simulink model "Sim_Saturation_iqctest1"  (Simulink 7.3)
settings: Solver=ode45  StartTime=0.0  StopTime=10.0  RelTol=1e-3
settings Model: Creator=MD710  LastModifiedBy=MD710
settings DebuggingCC: SaveWithParameterizedLinksMsg=none  SolverPrmCheckMsg=none  MultiTaskDSMMsg=warning  MultiTaskCondExecSysMsg=none  FcnCallInpInsideContextMsg=Enable All  StrictBusMsg=None
settings HardwareCC: TargetHWDeviceType=32-bit Generic
settings RTWCC: IncludeERTFirstTime=on
settings GRTTargetCC: TargetFcnLib=ansi_tfl_tmw.mat

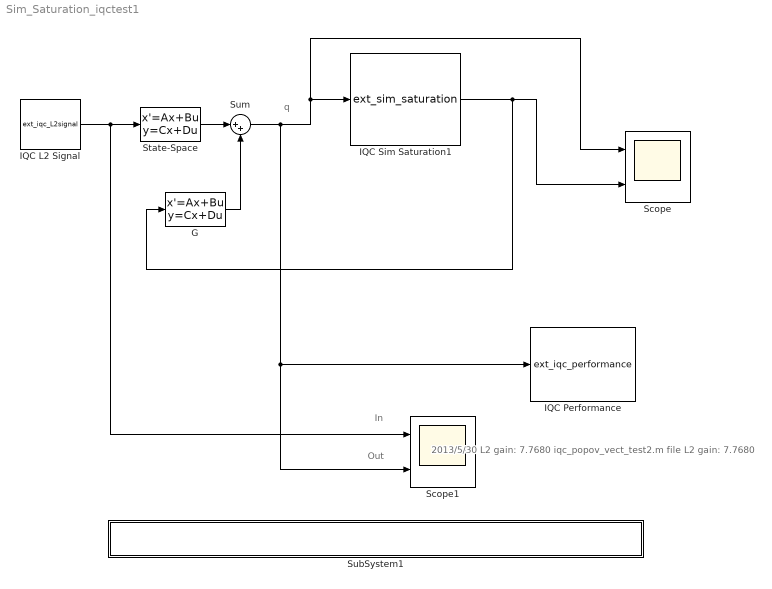
== system Sim_Saturation_iqctest1 ==
  note: q
  note: 2013/5/30 L2 gain: 7.7680
      | iqc_popov_vect_test2.m file L2 gain: 7.7680
  note: In
  note: Out
  G : StateSpace  A=[-0.37 0.20 0.15; -0.24 -0.65 0.51;0.09 -0.53 -0.60]  B="[-0.14 0; 0.11 -0.10;0   -0.83]"  C="[0.15   0    0;  0     0.8   0.4];"  D=[0 0;0 0]
  IQC L2 Signal : M-S-Function  FunctionName=ext_iqc_L2signal  Parameters=sig_size,sam_time,sig_type,tru_time,sig_amp,sig_fre,user_cus  mask(IQC L2 signal(ver:0.1)){sig_size=2, sam_time=0, sig_type=Step, tru_time=5, sig_amp=30, sig_fre=1, user_cus='2*exp(3*t)'}
      mask prompts: sig_size "Signal Dimension:(Default: 1)"; sam_time "Sample Time:(Default: 0)"; sig_type "Signal Type:"; tru_time "Truncation Time:"; sig_amp "Maximum Amplitude:"; sig_fre "Frequency:"; user_cus "Custom:"
      mask help:
      | Important:
      | In IQC procedure step (as commond iqc_gain_tbx, the task is get
      | L2 gain value), regardless of the user to choose which option (ex sine...),
      | here regarded as generalized L2 signal.
      mask StyleString: edit,edit,popup(Step|Square wave|Sine wave|Custom|Random|External),edit,edit,edit,edit
      mask CallbackString: ||iqc_block_cho(gcb,'L2signal_type')||||
      mask TabNameString: Main,Main,Simulation,Simulation,Simulation,Simulation,Simulation
      mask Display: plot(0:0.1:10,[sin(0:0.1:6.2) zeros(1,38)])
  IQC Performance : M-S-Function  FunctionName=ext_iqc_performance  Parameters=imp_met,save_lin_com,isiqcbode,fre_ran,uselmitool,lmi_par  mask(IQC Performance(ver:0.1)){imp_met=Calculation and Simulation, save_lin_com=off, isiqcbode=off, fre_ran='', uselmitool=lmilab, lmi_par=''}
      mask prompts: imp_met "Implementation Methods"; save_lin_com "Save the Linear File and Command File"; isiqcbode "Display IQC Bode Figure"; fre_ran "Frequency Range:(Default: empty)"; uselmitool "LMI Tool:"; lmi_par "Parameter:(if empty use define)"
      mask help:
      | Important:
      | In IQC toolbox calculate step (as commond iqc_gain_tbx, the task is get
      | L2 gain value), regardless of the user to connect any signal input(Even if
      | not a signal), here regarded as generalized L2 signal.
      |
      | Example 1: setlmioptions('',[0 200 0 0 777])
      | the block parameter is
      | LMI Tool: lmilab
      | Parameter:
      |        [0 200 0 0 777]
      |
      | Example 2: setlmioptions('yalmip','solver','sdpt3','verbose',1)
      | the block parameter is
      | LMI Tool: yalmip
      | Parameter:
      |        {'solver',sdpt3','verbose',1}
      mask Help:
      | <a href="matlab:doc abst_init_iqc;">abst_init_iqc</a>
      | <a href="matlab:doc setlmioptions;">setlmioptions</a>
      | <a href="matlab:doc iqc_gain_tbx;">iqc_gain_tbx</a>
      mask StyleString: popup(Calculation and Simulation|Only Calculation|Only Simulation),checkbox,checkbox,edit,popup(lmilab|yalmip),edit
      mask CallbackString: iqc_block_cho(gcb,'performance_imp')||iqc_block_cho(gcb,'performance_bodefre')|||
      mask TabNameString: Main,Main,Main,Main,LMI,LMI
      mask Display: fprintf('In -> Out \n performance \n L2 gain:\n%4.4f',7.768);
  IQC Sim Saturation1 : M-S-Function  FunctionName=ext_sim_saturation  Parameters=upp_lim,low_lim,sam_tim,iqc1,iqc1_pole,iqc1_ope,iqc1_out,iqc2,iqc2_out,iqc3,iqc3_out,iqc4,iqc4_sign,iqc4_out,iqc5,lis_rel  mask(IQC Sim Saturation(ver:0.1)){upp_lim=1, low_lim=-1, sam_tim=0, iqc1=off, iqc1_pole=[1], iqc1_ope=0 (shut off the Popov's IQC), iqc1_out='', iqc2=off, iqc2_out='', iqc3=off, iqc3_out='', iqc4=on, iqc4_sign='0', iqc4_out='', iqc5=on, lis_rel='out=iqc_tvscalar(in)'}
      mask prompts: upp_lim "Upper Limit:"; low_lim "Lower Limit:"; sam_tim "Sample Time:(Default: 0)"; iqc1 "iqc_monotonic(Input,Pole,Operator,1) (only for scalar input)"; iqc1_pole "Pole:(Default:[1])"; iqc1_ope "Operator:(Default: 0)"; iqc1_out "Output Variable:(Default: empty)"; iqc2 "iqc_sector(Input,0,1) (only for scalar input)"; iqc2_out "Output Variable:(Default: empty)"; iqc3 "iqc_popov(Input,0,1) (only for scalar input)"; iqc3_out "Output Variable:(Default: empty)"; iqc4 "iqc_popov_vect(Input,Sign)"; iqc4_sign "Sign:(Default: '0')"; iqc4_out "Output Variable:(Default: empty)"; iqc5 "Custom IQC"; lis_rel "List of IQC Relationships:"
      mask Help:
      | <a href="matlab:doc iqc_monotonic;">iqc_monotonic</a>
      | <a href="matlab:doc iqc_sector;">iqc_sector</a>
      | <a href="matlab:doc iqc_popov;">iqc_popov</a>
      | <a href="matlab:doc iqc_popov_vect;">iqc_popov_vect</a>
      mask StyleString: edit,edit,edit,checkbox,edit,popup(0 (shut off the Popov's IQC)|1 (turn on ther Popov's IQC)),edit,checkbox,edit,checkbox,edit,checkbox,popup('0'|'+'|'-'),edit,checkbox,edit
      mask CallbackString: |||iqc_block_cho(gcb,'sim_saturation_iqc1')||||iqc_block_cho(gcb,'sim_saturation_iqc2')||iqc_block_cho(gcb,'sim_saturation_iqc3')||iqc_block_cho(gcb,'sim_saturation_iqc4')|||iqc_block_cho(gcb,'sim_saturation_iqc5')|
      mask TabNameString: Simulation,Simulation,Simulation,Calculation,Calculation,Calculation,Calculation,Calculation,Calculation,Calculation,Calculation,Calculation,Calculation,Calculation,Calculation,Calculation
      mask Display: x=-10:10;for i=1:21;if x(i)>=-3 && x(i)<=3;y(i)=x(i);elseif x(i)<-3;y(i)=-3;elseif x(i)>3;y(i)=3;end;end;x1=zeros(1,11);y1=-5:1:5;y2=zeros(1,21);plot(x,y);plot(x1,y1);plot(x,y2)
  Scope : Scope  NumInputPorts=2
      settings: TimeRange=10  YMin=-2~-0.2  YMax=12~1.2
  Scope1 : Scope  NumInputPorts=2
      settings: YMin=-5~-5  YMax=5~5
  State-Space : StateSpace  A=[-1 0;0 -1]  B=[1 0;0 1]  C=[1 0;0 1]  D=[0 0;0 0]
  SubSystem1 : Subsystem  mask{filename=iqc_popov_vect_test2.m}
      mask init:
      | x_dir=which(filename);
      | x=x_dir;
      settings: OpenFcn=|
      | x_dir=which('iqc_popov_vect_test2.m');
      | x=x_dir;
      | edit(x);
      mask Display: disp(['MATLAB file: ' x]);
  Sum : Sum  Inputs=|++
  wires:
  IQC L2 Signal/1 -> Scope1/1, State-Space/1
  State-Space/1 -> Sum/1
  G/1 -> Sum/2
  Sum/1 -> IQC Sim Saturation1/1, Scope/1, IQC Performance/1, Scope1/2
  IQC Sim Saturation1/1 -> G/1, Scope/2

== system Sim_Saturation_iqctest1/SubSystem1 ==
